simulink model "blockdemo"  (Simulink 6.3)
settings: Solver=FixedStepDiscrete  StartTime=0.0  StopTime=16.0  RelTol=1e-3
InitFcn:
  | %% DSPBuilder Start
  | alt_dspbuilder_update_model(bdroot)
  | %% DSPBuilder End
libraries: allblocks_alteradspbuilder2 x5
settings Model: LastModifiedBy=delphick

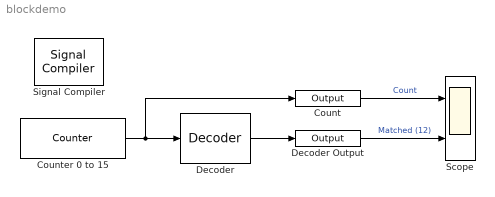
== system blockdemo ==
  Count : allblocks_alteradspbuilder2/Output  iofile=C:\workspace_clean\Documentation\DesignExamples\Tutorials\UnitBlocks\GateAndControl\Decoder\tb_blockdemo\blockdemo_Count.capture  BusType=Unsigned Integer  bwl=4  bwr=0  PORTTYPE=Output
  Counter 0 to 15 : allblocks_alteradspbuilder2/Counter  BusType=Unsigned Integer  bwl=4  bwr=0  use_modulo=on  modulo=16  SpecifyClock=off  direction=Increment  use_sload=off  use_sset=off  svalue=1  use_ena=off  use_sclr=off
  Decoder : allblocks_alteradspbuilder2/Decoder  BusType=Unsigned Integer  bwl=4  bwr=2  registered=on  value=12
  Decoder Output : allblocks_alteradspbuilder2/Output  iofile=C:\workspace_clean\Documentation\DesignExamples\Tutorials\UnitBlocks\GateAndControl\Decoder\tb_blockdemo\blockdemo_Decoder+Output.capture  BusType=Single Bit  bwl=8  bwr=0  PORTTYPE=Output
  Scope : Scope  NumInputPorts=2
      settings: TimeRange=16  YMin=0~-2  YMax=16~2
  Signal Compiler : allblocks_alteradspbuilder2/Signal Compiler  DeviceFamily=Stratix IV  DeviceName=AUTO  EnableSignalTap=off  SignalTapDepth=128  UseBoardBlock=off  StpUseDefaultClock=on  StpClock=clock
  wires:
  Counter 0 to 15/1 -> Count/1, Decoder/1
  Decoder/1 -> Decoder Output/1
  Count/1 -> Scope/1  "Count"
  Decoder Output/1 -> Scope/2  "Matched (12)"
